simulink model "Problem_7"  (R2020b)
settings: Solver=VariableStepAuto  StartTime=0.0  StopTime=10.0  RelTol=1e-3
settings Model: Creator=HP  LastModifiedBy=HP

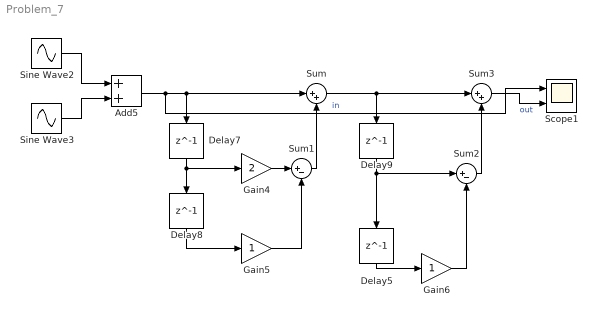
== system Problem_7 ==
  Add5 : Sum
  Delay{5,7..9} (4 alike) : Delay  DelayLength=1
  Gain4 : Gain  Gain=2
  Gain5 : Gain
  Gain6 : Gain
  Scope1 : Scope  NumInputPorts=2
  Sine Wave2 : Sin  SampleTime=0
  Sine Wave3 : Sin  Amplitude=0.5  Frequency=50  SampleTime=0
  Sum : Sum  Inputs=|++
  Sum1 : Sum  Inputs=|+-
  Sum2 : Sum  Inputs=|+-
  Sum3 : Sum  Inputs=|++
  wires:
  Delay5/1 -> Gain6/1
  Sum2/1 -> Sum3/2
  Delay9/1 -> Sum2/1, Delay5/1
  Gain4/1 -> Sum1/1
  Sine Wave2/1 -> Add5/1
  Gain5/1 -> Sum1/2
  Sum/1 -> Delay9/1, Sum3/1
  Delay8/1 -> Gain5/1
  Gain6/1 -> Sum2/2
  Add5/1 -> Scope1/1, Delay7/1, Sum/1  "in"
  Sum1/1 -> Sum/2
  Delay7/1 -> Delay8/1, Gain4/1
  Sine Wave3/1 -> Add5/2
  Sum3/1 -> Scope1/2  "out"
